simulink model "Lazo_Abierto"  (R2021a)
settings: Solver=ode45  StartTime=0.0  StopTime=t_sim  RelTol=1e-3
values from neighbouring files (symbols this model uses):
  A_1_low = 0.50    (= 0.5)    [Main_Lazo_Abierto.m]
  A_1_mid = A_1_max - A_1_min    (= 0.79)    [Main_Lazo_Abierto.m]
  A_1_min = 0.21    [Main_Lazo_Abierto.m]
  A_1_upp = 1    [Main_Lazo_Abierto.m]
  alfa = 0.034    [ParametrosModelo.m]
  beta = 1.33    [ParametrosModelo.m]
  CO2s = yCO2 /HenryCO2    (= 0.666844491864)    [ParametrosModelo.m]
  delta = 0.89    [ParametrosModelo.m]
  Estrategia = 1    [Main_Lazo_Abierto.m]
  G_1_low = 0.30    (= 0.3)    [Main_Lazo_Abierto.m]
  G_1_mid = G_1_max - G_1_min    (= 0.4)    [Main_Lazo_Abierto.m]
  G_1_min = 0.2    [Main_Lazo_Abierto.m]
  G_1_upp = 0.50    (= 0.5)    [Main_Lazo_Abierto.m]
  gamma = 0.603    [ParametrosModelo.m]
  Henry = 26.409    [ParametrosModelo.m]
  ks1 = 1    [ParametrosModelo.m]
  kx1 = 0.49    [ParametrosModelo.m]
  mu_set = 0.13    [ParametrosModelo.m]
  N_1_low = 0    [Main_Lazo_Abierto.m]
  N_1_max = 300    [Main_Lazo_Abierto.m]
  N_1_min = 300    [Main_Lazo_Abierto.m]
  N_1_upp = 0.30    (= 0.3)    [Main_Lazo_Abierto.m]
  PI_Kd = 0    [Main_Lazo_Abierto.m]
  PI_Kd_2 = 0    [Main_Lazo_Abierto.m]
  PI_Ki = 1163.22932064265    (= 1163.22932064)    [Main_Lazo_Abierto.m]
  PI_Ki_2 = 0.06    [Main_Lazo_Abierto.m]
  PI_Kp = 1.87082881181595    (= 1.87082881182)    [Main_Lazo_Abierto.m]
  PI_Kp_2 = 13.0    (= 13)    [Main_Lazo_Abierto.m]
  Si = 500    [ParametrosModelo.m]
  spO2 = 0.3*O2s    [Main_Lazo_Abierto.m]
  Ts = 0.0166666666667    [CondicionesIniciales.mat]    (also in Main_Lazo_Abierto.m)
  u_1_low = 0    [Main_Lazo_Abierto.m]
  u_1_upp = 1    [Main_Lazo_Abierto.m]
  v0 = 0.3    [CondicionesIniciales.mat]    (also in Main_Lazo_Abierto.m)
  V_Stop = 3    [Main_Lazo_Abierto.m]
  x0 = 5    [CondicionesIniciales.mat]    (also in Floripa004.m = C_iniciales; Main_Lazo_Abierto.m)
undefined symbols (not defined in the file or in its folder): magnitude
libraries: simulink x7, pid_lib x1
settings Model: Creator=Bastiacito88  LastModifiedBy=dnavalos
settings SolverCC: AlgebraicLoopSolver=TrustRegion
settings DataIOCC: ReturnWorkspaceOutputs=off
settings DebuggingCC: SFMachineParentedDataDiag=warning  ArithmeticOperatorsInVariantConditions=warning
settings SFSimCC: SimUseLocalCustomCode=off  CustomCodeUndefinedFunction=UseInterfaceOnly
settings RTWCC: RTWUseLocalCustomCode=off

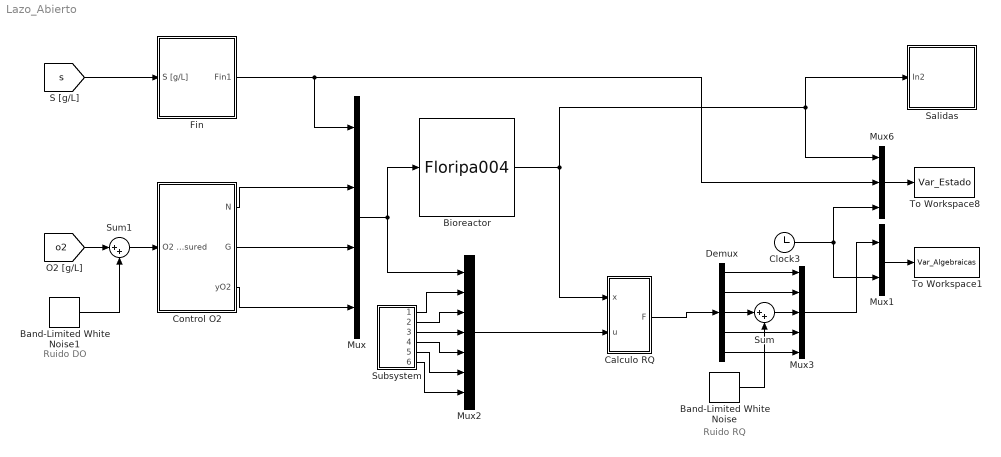
== system Lazo_Abierto ==
  note: Ruido DO
  note: Ruido RQ
  Band-Limited White Noise : simulink/Sources/Band-Limited White Noise  Cov=sigma_RQ  Ts=Ts  seed=[23341]
  Band-Limited White Noise1 : simulink/Sources/Band-Limited White Noise  Cov=sigma_DO  Ts=Ts  seed=[23341]
  Bioreactor : S-Function  FunctionName=Floripa004  SFunctionDeploymentMode=off  EnableBusSupport=off
      mask Display: image('Biored.jpg');
  Calculo RQ : MATLAB Function  TreatAsAtomicUnit=on
  Clock3 : Clock
  Control O2 : Subsystem
  Demux : Demux  Outputs=5
  Fin : Subsystem
      mask Display: image('Bomba.jpg');
  Mux : Mux
  Mux1 : Mux  Inputs=2
  Mux2 : Mux  Inputs=7
  Mux3 : Mux  Inputs=5
  Mux6 : Mux  Inputs=3
  Salidas : Subsystem
  Subsystem : Subsystem
  Sum : Sum  Inputs=|++
  Sum1 : Sum  Inputs=|++
  To Workspace1 : ToWorkspace  VariableName=Var_Algebraicas  SampleTime=-1
  To Workspace8 : ToWorkspace  VariableName=Var_Estado  SampleTime=-1
  wires:
  Subsystem/6(Out6) -> Mux2/7
  Control O2/3(yO2) -> Mux/4
  Mux1/1 -> To Workspace1/1
  Clock3/1 -> Mux6/3, Mux1/2
  Control O2/1(N) -> Mux/2
  Subsystem/4(Out4) -> Mux2/5
  Subsystem/5(Out5) -> Mux2/6
  Calculo RQ/1(F) -> Demux/1
  Bioreactor/1 -> Calculo RQ/1(x), Mux6/1, Salidas/1(In2)
  Subsystem/1(Out1) -> Mux2/2
  [s] -> Fin/1(S [g/L])
  Subsystem/2(Out2) -> Mux2/3
  Fin/1(Fin1) -> Mux6/2, Mux/1
  Mux2/1 -> Calculo RQ/2(u)
  Control O2/2(G) -> Mux/3
  Subsystem/3(Out3) -> Mux2/4
  Mux6/1 -> To Workspace8/1
  Mux/1 -> Mux2/1, Bioreactor/1
  Mux3/1 -> Mux1/1
  Demux/1 -> Mux3/1
  Demux/2 -> Mux3/2
  Demux/4 -> Mux3/4
  Demux/5 -> Mux3/5
  Demux/3 -> Sum/1
  Band-Limited White Noise/1 -> Sum/2
  Sum/1 -> Mux3/3
  Sum1/1 -> Control O2/1(O2 measured)
  [o2] -> Sum1/1
  Band-Limited White Noise1/1 -> Sum1/2

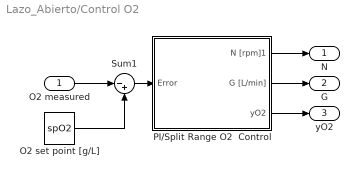
== system Lazo_Abierto/Control O2 ==
  O2 measured : Inport
  O2 set point [g/L] : Constant  Value=spO2
  PI/Split Range O2  Control : Subsystem
  Sum1 : Sum  Inputs=|-+
  N : Outport  VectorParamsAs1DForOutWhenUnconnected=off
  G : Outport  Port=2  VectorParamsAs1DForOutWhenUnconnected=off
  yO2 : Outport  Port=3  VectorParamsAs1DForOutWhenUnconnected=off
  wires:
  PI/Split Range O2  Control/1(N [rpm]1) -> N/1
  PI/Split Range O2  Control/2(G [L/min]) -> G/1
  O2 measured/1 -> Sum1/1
  O2 set point [g/L]/1 -> Sum1/2
  PI/Split Range O2  Control/3("yO2 ") -> yO2/1
  Sum1/1 -> PI/Split Range O2  Control/1(Error)

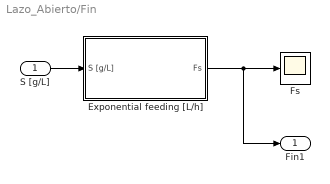
== system Lazo_Abierto/Fin ==
  S [g/L] : Inport
  Exponential feeding [L/h] : Subsystem
  Fs : Scope
  Fin1 : Outport  VectorParamsAs1DForOutWhenUnconnected=off
  wires:
  S [g/L]/1 -> Exponential feeding [L/h]/1(S [g/L])
  Exponential feeding [L/h]/1(Fs) -> Fin1/1, Fs/1

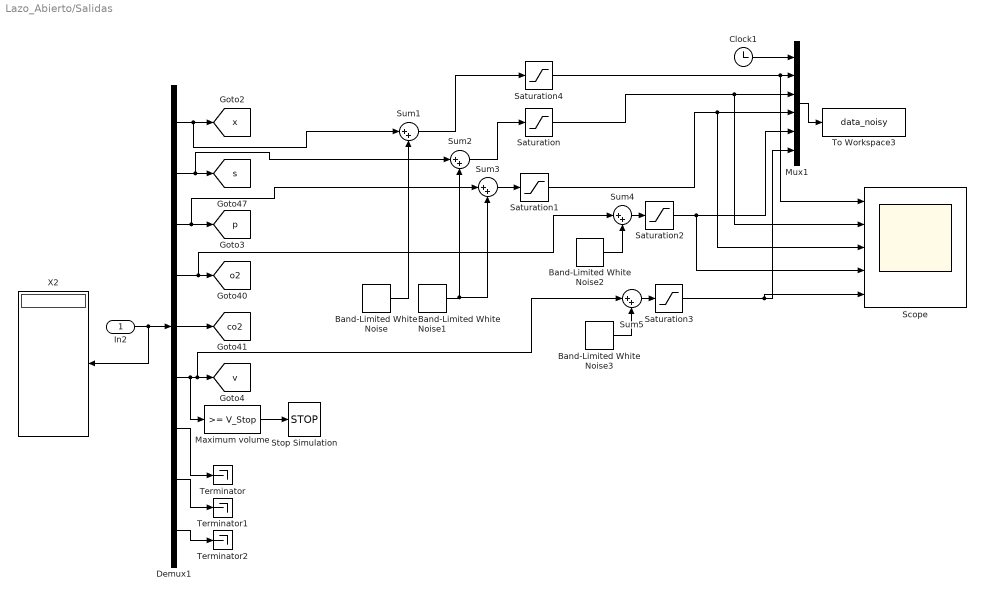
== system Lazo_Abierto/Salidas ==
  In2 : Inport
  Band-Limited White Noise : simulink/Sources/Band-Limited White Noise  Cov=[10]  Ts=0.2  seed=[23341]
  Band-Limited White Noise1 : simulink/Sources/Band-Limited White Noise  Cov=[1e-4]  Ts=0.2  seed=[23341]
  Band-Limited White Noise2 : simulink/Sources/Band-Limited White Noise  Cov=[1e-8]  Ts=0.2  seed=[23341]
  Band-Limited White Noise3 : simulink/Sources/Band-Limited White Noise  Cov=[0.01]  Ts=0.2  seed=[23341]
  Clock1 : Clock
  Demux1 : Demux  Outputs=9
  Maximum volume : simulink/Logic and Bit Operations/Compare To Constant  relop=>=  const=V_Stop  OutDataTypeStr=boolean
  Mux1 : Mux  Inputs=6
  Saturation{,1..4} (5 alike) : Saturate  UpperLimit=inf  LowerLimit=0
  Scope : Scope  NumInputPorts=5
  Stop Simulation : Stop
  Sum{1..5} (5 alike) : Sum  Inputs=|++
  Terminator : Terminator
  Terminator1 : Terminator
  Terminator2 : Terminator
  To Workspace3 : ToWorkspace  VariableName=data_noisy  SampleTime=1
  X2 : Display
  tag scope: co2=global, o2=global, p=global, s=global, v=global, x=global
  wires:
  Demux1/9 -> Terminator2/1
  Demux1/8 -> Terminator1/1
  Demux1/5 -> [co2]
  Demux1/7 -> Terminator/1
  Maximum volume/1 -> Stop Simulation/1
  In2/1 -> X2/1, Demux1/1
  Sum5/1 -> Saturation3/1
  Band-Limited White Noise3/1 -> Sum5/2
  Saturation4/1 -> Scope/1, Mux1/2
  Sum3/1 -> Saturation1/1
  Clock1/1 -> Mux1/1
  Demux1/4 -> Sum4/1, [o2]
  Sum4/1 -> Saturation2/1
  Demux1/6 -> Sum5/1, [v], Maximum volume/1
  Saturation1/1 -> Scope/3, Mux1/4
  Sum2/1 -> Saturation/1
  Saturation/1 -> Scope/2, Mux1/3
  Demux1/3 -> Sum3/1, [p]
  Saturation2/1 -> Scope/4, Mux1/5
  Sum1/1 -> Saturation4/1
  Demux1/1 -> Sum1/1, [x]
  Demux1/2 -> Sum2/1, [s]
  Band-Limited White Noise/1 -> Sum1/2
  Saturation3/1 -> Scope/5, Mux1/6
  Mux1/1 -> To Workspace3/1
  Band-Limited White Noise2/1 -> Sum4/2
  Band-Limited White Noise1/1 -> Sum3/2, Sum2/2

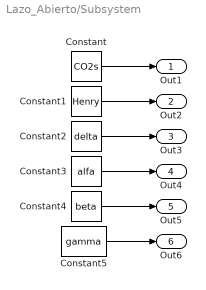
== system Lazo_Abierto/Subsystem ==
  Constant : Constant  Value=CO2s
  Constant1 : Constant  Value=Henry
  Constant2 : Constant  Value=delta
  Constant3 : Constant  Value=alfa
  Constant4 : Constant  Value=beta
  Constant5 : Constant  Value=gamma
  Out1 : Outport  VectorParamsAs1DForOutWhenUnconnected=off
  Out2 : Outport  Port=2  VectorParamsAs1DForOutWhenUnconnected=off
  Out3 : Outport  Port=3  VectorParamsAs1DForOutWhenUnconnected=off
  Out4 : Outport  Port=4  VectorParamsAs1DForOutWhenUnconnected=off
  Out5 : Outport  Port=5  VectorParamsAs1DForOutWhenUnconnected=off
  Out6 : Outport  Port=6  VectorParamsAs1DForOutWhenUnconnected=off
  wires:
  Constant2/1 -> Out3/1
  Constant3/1 -> Out4/1
  Constant1/1 -> Out2/1
  Constant4/1 -> Out5/1
  Constant5/1 -> Out6/1
  Constant/1 -> Out1/1

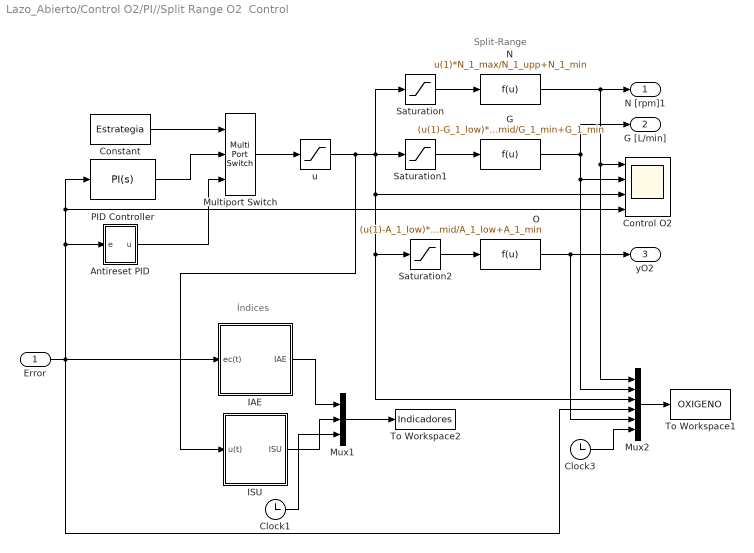
== system Lazo_Abierto/Control O2/PI//Split Range O2  Control ==
  note: Índices
  note: Split-Range
  Error : Inport
  Antireset PID : Subsystem  mask(Antireset PID){G=PI_Kp_2, ti=PI_Ki_2, td=PI_Kd_2, a=0.5, U=1, L=0}
      mask prompts: G "Controller Gain"; ti "Integral Time Constant"; td "Derivative Time Constant"; a "Alpha"; U "Saturation Upper Limit"; L "Saturation Lower Limit"
      mask help: Enter expression for Controller Gain, Integral Time Constant, Derivative Time Constant, Alpha Constant, Saturation Upper Constant, and Saturation Lower Constant terms.
  Clock1 : Clock
  Clock3 : Clock
  Constant : Constant  Value=Estrategia
  Control O2 : Scope  NumInputPorts=4
  G : Fcn  Expr=(u(1)-G_1_low)*G_1_mid/G_1_min+G_1_min
  IAE : Subsystem
  ISU : Subsystem
  Multiport Switch : MultiPortSwitch  Inputs=2
  Mux1 : Mux  Inputs=3
  Mux2 : Mux  Inputs=6
  N : Fcn  Expr=u(1)*N_1_max/N_1_upp+N_1_min
  O : Fcn  Expr=(u(1)-A_1_low)*A_1_mid/A_1_low+A_1_min
  PID Controller : pid_lib/PID Controller  Controller=PI  Form=Parallel  TimeDomain=Continuous-time  UseExternalTs=off  SampleTime=-1  IntegratorMethod=Forward Euler  FilterMethod=Forward Euler  ControllerParametersSource=internal  P=PI_Kp  I=PI_Ki  D=PI_Kd  UseFilter=on  N=479.898765366224  TunerSelectOption=Transfer Function Based (PID Tuner App)  InitialConditionSource=internal  InitialConditionForIntegrator=-48.255  InitialConditionForFilter=0  DifferentiatorICPrevScaledInput=0  ExternalReset=none  TrackingMode=off  Kt=1  LimitOutput=on  SatLimitsSource=internal  UpperSaturationLimit=1  LowerSaturationLimit=0  LinearizeAsGain=off  AntiWindupMode=back-calculation  Kb=1  POutMin=[]  POutMax=[]  IOutMin=[]  IOutMax=[]  DOutMin=[]  DOutMax=[]  NOutMin=[]  NOutMax=[]  SumOutMin=[]  SumOutMax=[]  SaturationOutMin=[]  SaturationOutMax=[]  PParamMin=[]  PParamMax=[]  IParamMin=[]  IParamMax=[]  DParamMin=[]  DParamMax=[]  NParamMin=[]  NParamMax=[]  KbParamMin=[]  KbParamMax=[]  KtParamMin=[]  KtParamMax=[]  KbOutMin=[]  KbOutMax=[]  KtOutMin=[]  KtOutMax=[]  IntegratorOutMin=[]  IntegratorOutMax=[]  FilterOutMin=[]  FilterOutMax=[]  SumI1OutMin=[]  SumI1OutMax=[]  SumI2OutMin=[]  SumI2OutMax=[]  SumI3OutMin=[]  SumI3OutMax=[]  SumI4OutMin=[]  SumI4OutMax=[]  SumDOutMin=[]  SumDOutMax=[]  DifferentiatorOutMin=[]  DifferentiatorOutMax=[]  FilterDiffOutCoefMin=[]  FilterDiffOutCoefMax=[]  ReciprocalOutMin=[]  ReciprocalOutMax=[]  SumDenOutMin=[]  SumDenOutMax=[]  SumNumOutMin=[]  SumNumOutMax=[]  DivideOutMin=[]  DivideOutMax=[]  UdiffTsProdOutMin=[]  UdiffTsProdOutMax=[]  NTsProdOutMin=[]  NTsProdOutMax=[]  UintegralTsProdOutMin=[]  UintegralTsProdOutMax=[]  UngainTsProdOutMin=[]  UngainTsProdOutMax=[]  IntegratorContinuousStateAttributes=''  IntegratorStateMustResolveToSignalObject=off  IntegratorRTWStateStorageClass=Auto  FilterContinuousStateAttributes=''  FilterStateMustResolveToSignalObject=off  FilterRTWStateStorageClass=Auto  ParallelPVariant=InternalParameters  IdealPVariant=Disabled  IVariant=InternalParameters  DVariant=Disabled  IntegratorVariant=Continuous  SatVariant=Enabled  AWVariant=BackCalculation  PCopyVariant=Disabled  TRVariant=Disabled  FdbkBlocksVariant=Forward  IdealPFdbkVariant=Disabled  SatFdbkVariant=Disabled  DerivativeFilterVariant=Disabled  NVariant=Disabled  NCopyVariant=Disabled_SignalSpec  FilterICVariant=Disabled  IntegratorICVariant=InternalICs  ExternalResetVariant=Disabled  TRSumVariant=Passthrough  SumFdbkVariant=Disabled  SumVariant=Sum_PI  TsampFilterVariant=InternalTs  TsampNgainVariant=Passthrough  TsampIntegralVariant=Passthrough  ExternalSaturationOutDataTypeStr=Inherit: Same as second input
  Saturation : Saturate  UpperLimit=N_1_upp  LowerLimit=N_1_low
  Saturation1 : Saturate  UpperLimit=G_1_upp  LowerLimit=G_1_low
  Saturation2 : Saturate  UpperLimit=A_1_upp  LowerLimit=A_1_low
  To Workspace1 : ToWorkspace  VariableName=OXIGENO  SampleTime=-1
  To Workspace2 : ToWorkspace  VariableName=Indicadores  SampleTime=-1
  u : Saturate  UpperLimit=u_1_upp  LowerLimit=u_1_low
  N [rpm]1 : Outport  VectorParamsAs1DForOutWhenUnconnected=off
  G [L/min] : Outport  Port=2  VectorParamsAs1DForOutWhenUnconnected=off
  "yO2 " : Outport  Port=3  VectorParamsAs1DForOutWhenUnconnected=off
  wires:
  Saturation2/1 -> O/1
  Constant/1 -> Multiport Switch/1
  Clock3/1 -> Mux2/6
  N/1 -> N [rpm]1/1, Mux2/1, Control O2/1
  Multiport Switch/1 -> u/1
  ISU/1(ISU) -> Mux1/2
  IAE/1(IAE) -> Mux1/1
  Clock1/1 -> Mux1/3
  Mux1/1 -> To Workspace2/1
  Mux2/1 -> To Workspace1/1
  PID Controller/1 -> Multiport Switch/2
  Saturation1/1 -> G/1
  Saturation/1 -> N/1
  O/1 -> Mux2/5, "yO2 "/1
  Antireset PID/1(u) -> Multiport Switch/3
  u/1 -> ISU/1(u(t)), Saturation/1, Saturation1/1, Mux2/3, Saturation2/1, Control O2/3
  G/1 -> G [L/min]/1, Mux2/2, Control O2/2
  Error/1 -> PID Controller/1, Control O2/4, Antireset PID/1(e), Mux2/4, IAE/1(ec(t))

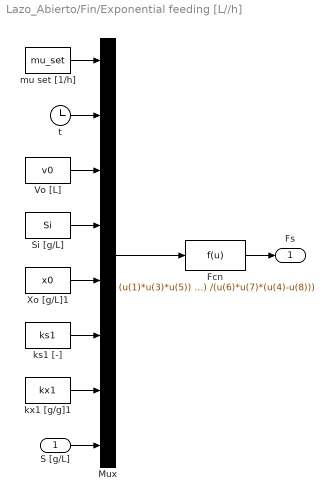
== system Lazo_Abierto/Fin/Exponential feeding [L//h] ==
  S [g/L] : Inport
  Fcn : Fcn  Expr=(u(1)*u(3)*u(5)) *(exp(u(1)*u(2))) /(u(6)*u(7)*(u(4)-u(8)))
  Mux : Mux  Inputs=8
  Si [g/L] : Constant  Value=Si
  Vo [L] : Constant  Value=v0
  Xo [g/L]1 : Constant  Value=x0
  ks1 [-] : Constant  Value=ks1
  kx1 [g/g]1 : Constant  Value=kx1
  mu set [1/h] : Constant  Value=mu_set
  t : Clock
  Fs : Outport  VectorParamsAs1DForOutWhenUnconnected=off
  wires:
  Si [g/L]/1 -> Mux/4
  t/1 -> Mux/2
  ks1 [-]/1 -> Mux/6
  Fcn/1 -> Fs/1
  Xo [g/L]1/1 -> Mux/5
  kx1 [g/g]1/1 -> Mux/7
  S [g/L]/1 -> Mux/8
  Vo [L]/1 -> Mux/3
  Mux/1 -> Fcn/1
  mu set [1/h]/1 -> Mux/1

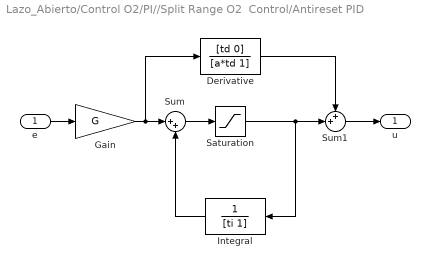
== system Lazo_Abierto/Control O2/PI//Split Range O2  Control/Antireset PID ==
  e : Inport
  Derivative : TransferFcn  Numerator=[td 0]  Denominator=[a*td 1]
  Gain : Gain  Gain=G  SaturateOnIntegerOverflow=on  OutDataTypeStr=Inherit: Same as input  ParamDataTypeStr=Inherit: Same as input
  Integral : TransferFcn  Denominator=[ti 1]
  Saturation : Saturate  UpperLimit=U  LowerLimit=L
  Sum : Sum  Inputs=|++  InputSameDT=on  SaturateOnIntegerOverflow=on  OutDataTypeStr=Inherit: Same as first input
  Sum1 : Sum  Inputs=++|  InputSameDT=on  SaturateOnIntegerOverflow=on  OutDataTypeStr=Inherit: Same as first input
  u : Outport  VectorParamsAs1DForOutWhenUnconnected=off
  wires:
  Derivative/1 -> Sum1/1
  Sum1/1 -> u/1
  Saturation/1 -> Integral/1, Sum1/2
  e/1 -> Gain/1
  Integral/1 -> Sum/2
  Sum/1 -> Saturation/1
  Gain/1 -> Derivative/1, Sum/1

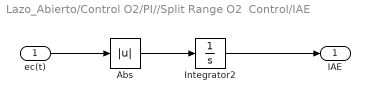
== system Lazo_Abierto/Control O2/PI//Split Range O2  Control/IAE ==
  ec(t) : Inport
  Abs : Abs
  Integrator2 : Integrator
  IAE : Outport  VectorParamsAs1DForOutWhenUnconnected=off
  wires:
  Abs/1 -> Integrator2/1
  ec(t)/1 -> Abs/1
  Integrator2/1 -> IAE/1

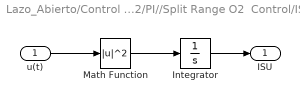
== system Lazo_Abierto/Control O2/PI//Split Range O2  Control/ISU ==
  u(t) : Inport
  Integrator : Integrator
  Math Function : Math  Operator=magnitude^2  SignedPower=on  SaturateOnIntegerOverflow=on
  ISU : Outport  VectorParamsAs1DForOutWhenUnconnected=off
  wires:
  Integrator/1 -> ISU/1
  u(t)/1 -> Math Function/1
  Math Function/1 -> Integrator/1

== matlab function Lazo_Abierto/Calculo RQ ==
  data: x input; F output; u input
function F = fcn(x, u)

% States
O2  =  x(4);                                 % Dissolved O2,     [g/L]
CO2 =  x(5);                                % Dissolved CO2,    [g/L]

% Parameters
MM_CO2 = 44.01;                       %Molar Mass CO2 [g/mol]
MM_O2 = 15.99*2;                     %Molar Mass CO2 [g/mol]

% Inputs
N   = u(2);
G   = u(3);
yo2 = u(4); 
CO2s = u(5);
Henry = u(6);
delta = u(7);

% Control law parameters
alfa = u(8);                                % [1/h], R2
beta = u(9);                               % [1/h], R2
gamma = u(10);                       % [1/h], R2

% Ecuaciones algebraicas
klao2 = 5*alfa*(N^beta)*(G^gamma); % Mass transfer coefficient for O2,[1/h]
klaco2 = delta*klao2;
CER = klaco2 *(CO2-CO2s)/MM_CO2;
OUR = klao2*(yo2/Henry-O2)/MM_O2;
RQ = CER/OUR;

F = [klao2; klaco2; RQ; CER; OUR];
